simulink model "plasmaModel"  (R2014a)
settings: Solver=ode3  StartTime=time(1)  StopTime=1  FixedStep=0.0005  RelTol=1e-3
values from neighbouring files (symbols this model uses):
  Ipl = interp1(dato.IplOldMis.x,dato.IplOldMis.y,time)    [main.m]    (also in main35965.m = interp1(dato.IPLmis.x,dato.IPLmis.y,time); main36634.m = interp1(dato.IPLmis.x,dato.IPLmis.y,time))
  Lp0 = 2*10^(-6)    (= 2e-06)    [globalVar.m]
  Mpt0 = 110*10^(-6)    (= 0.00011)    [globalVar.m]    (also in main35965.m = 0.000107; main36634.m = 0.000107)
  Mpv0 = 80*10^(-6)    (= 8e-05)    [globalVar.m]    (also in main35965.m = 7.5e-05; main36634.m = 7.5e-05)
  Rp = 2.5e-6    (= 2.5e-06)    [main.m]    (also in main35965.m = 5e-06; main36634.m = 5e-06)
settings Model: Creator=mateusz  LastModifiedBy=mateusz

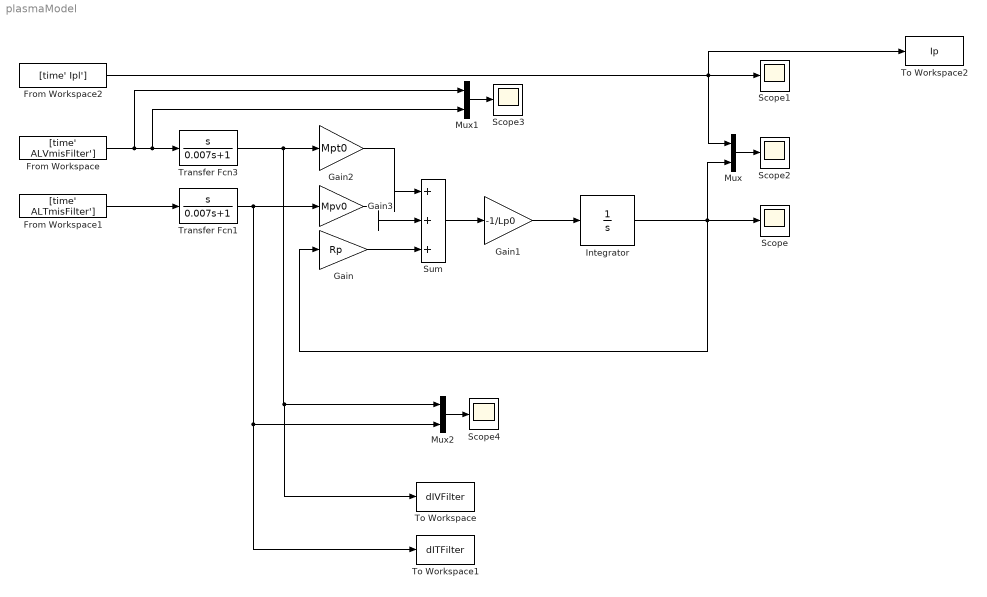
== system plasmaModel ==
  From Workspace : FromWorkspace  VariableName=[time' ALVmisFilter']  SampleTime=0
  From Workspace1 : FromWorkspace  VariableName=[time' ALTmisFilter']  SampleTime=0
  From Workspace2 : FromWorkspace  VariableName=[time' Ipl']  SampleTime=0
  Gain : Gain  Gain=Rp
  Gain1 : Gain  Gain=-1/Lp0
  Gain2 : Gain  Gain=Mpt0
  Gain3 : Gain  Gain=Mpv0
  Integrator : Integrator  InitialCondition=Ipl(1)
  Mux : Mux  Inputs=2
  Mux1 : Mux  Inputs=2
  Mux2 : Mux  Inputs=2
  Scope{,1..4} (5 alike) : Scope
      Scope2 settings: SaveName=ScopeData2
      Scope3 settings: SaveName=ScopeData3
      Scope4 settings: SaveName=ScopeData4
  Sum : Sum  Inputs=|+++
  To Workspace : ToWorkspace  VariableName=dIVFilter  SaveFormat=Timeseries  SampleTime=-1
  To Workspace1 : ToWorkspace  VariableName=dITFilter  SaveFormat=Timeseries  SampleTime=-1
  To Workspace2 : ToWorkspace  VariableName=Ip  SaveFormat=Timeseries  SampleTime=-1
  Transfer Fcn1 : TransferFcn  Numerator=[1 0]  Denominator=[0.007 1]
  Transfer Fcn3 : TransferFcn  Numerator=[1 0]  Denominator=[0.007 1]
  wires:
  Integrator/1 -> Mux/2, Scope/1, Gain/1
  Gain1/1 -> Integrator/1
  Sum/1 -> Gain1/1
  Gain/1 -> Sum/3
  Gain2/1 -> Sum/1
  Gain3/1 -> Sum/2
  Transfer Fcn3/1 -> Gain2/1, To Workspace/1, Mux2/1
  Transfer Fcn1/1 -> To Workspace1/1, Mux2/2, Gain3/1
  Mux/1 -> Scope2/1
  Mux1/1 -> Scope3/1
  From Workspace/1 -> Transfer Fcn3/1, Mux1/2, Mux1/1
  From Workspace2/1 -> To Workspace2/1, Mux/1, Scope1/1
  From Workspace1/1 -> Transfer Fcn1/1
  Mux2/1 -> Scope4/1
